simulink model "SIMULINK_02_HOMEWORK_INVERSE_IDENTIFICATION_SANTIAGO_GARCIA"  (R2020a)
settings: Solver=FixedStepAuto  StartTime=0.0  StopTime=150  FixedStep=0.01  RelTol=1e-2
libraries: simulink x1
settings Model: Creator=elkin  LastModifiedBy=USUARIO

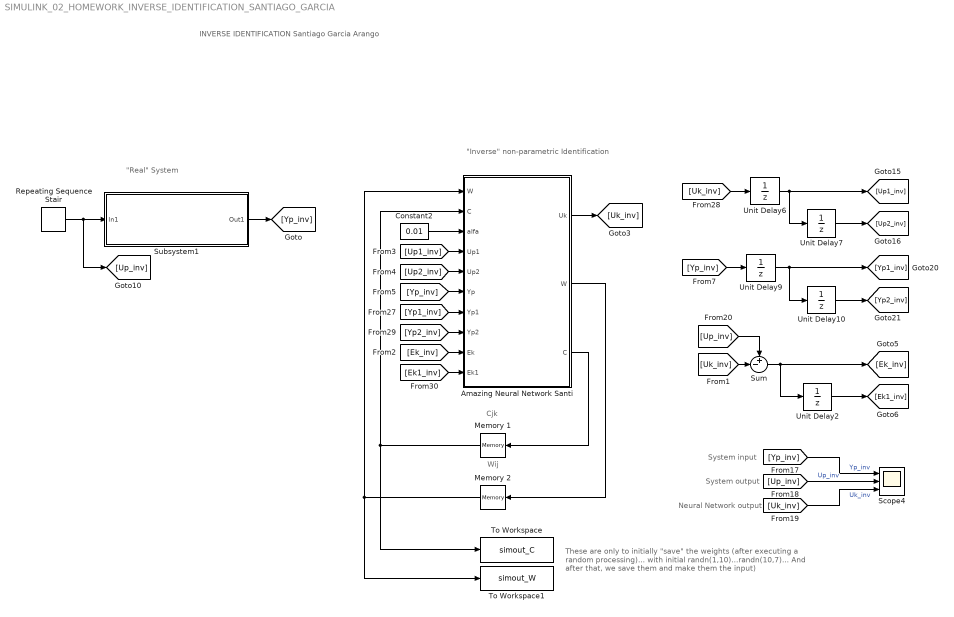
== system SIMULINK_02_HOMEWORK_INVERSE_IDENTIFICATION_SANTIAGO_GARCIA ==
  note: These are only to initially "save" the weights (after executing a random processing)... with initial randn(1,10)...randn(10,7)...
      | And after that,  we save them and make them the input)
  note: "Real" System
  note: INVERSE IDENTIFICATION
      | Santiago Garcia Arango
  note: "Inverse" non-parametric Identification
  note: Cjk
  note: Wij
  note: System input
  note: System output
  note: Neural Network output
  " Memory 2" : Memory  InitialCondition=[0.160168468969978,1.21353137879989,-1.56291773173372,0.929169980143353,0.695994193594052,-1.34686510381095,-0.289653748521687;0.421933175617497,0.436877187593544,0.666165671349512,0.137541063195606,-1.07644666007559,0.241226964817676,2.09884854078536;-0.0777054777653791,1.26008707442584,0.0176636587033483,0.0774381989337176,0.329568098519725,0.923600106862029,0.0294305745416468;-1.40499547474677,-0.342765649438291,-1.04188122704995,0.851174491843777,0.544969535049168,0.739674158347271,1.10397908720867;-0.0112601196223381,-0.768799183156363,-0.315486308406169,1.21256202395209,0.173176764089594,-0.178755445313924,-0.334973975015624;-0.556892652341610,0.141789370522390,-1.73598081128122,-0.978665689175691,0.645874102776012,-2.00118746022715,-0.989945469292243;-1.21745485974872,1.36268884465170,0.447025596332749,1.33569188423369,-1.15629544144397,-1.04648278411230,0.648907387350675;-0.0124054854051064,1.27274230512064,-0.172396006495970,-1.20850709692038,1.00898576278285,0.264634046236538,1.00048012001628;-0.195144705340148,-0.142308239828302,1.63129654132556,-1.07404750027954,0.113599563813982,0.811933866909450,1.80624743610141;0.273984746210026,-0.638527379745420,-1.35171776281153,-0.664986054870598,0.737505072399746,0.532586026418463,-0.586211714839106]
  Amazing Neural Network Santi : MATLAB Function  TreatAsAtomicUnit=on
  Constant2 : Constant  Value=0.01
  Memory 1 : Memory  InitialCondition=[-2.03120000000000,1.12670000000000,0.0650000000000000,-1.22620000000000,-0.274400000000000,-0.965500000000000,0.418700000000000,0.122100000000000,-0.0491000000000000,0.714800000000000]
  Repeating Sequence Stair : simulink/Sources/Repeating Sequence Stair  OutValues=[0 0.2 0 0.4 0.8 0.4 1].'  tsamp=15  OutMin=[]  OutMax=[]  OutDataTypeStr=double  OutputDataTypeScalingMode=double  OutDataType=fixdt(0,8)  ConRadixGroup=Best Precision: Vector-wise  OutScaling=2^-12
  Scope4 : Scope  NumInputPorts=3
  Subsystem1 : Subsystem
  Sum : Sum  Inputs=+-|
  To Workspace : ToWorkspace  VariableName=simout_C  SaveFormat=Timeseries  SampleTime=-1
  To Workspace1 : ToWorkspace  VariableName=simout_W  SaveFormat=Timeseries  SampleTime=-1
  Unit Delay{2,6..7,9..10} (5 alike) : UnitDelay  SampleTime=-1  HasFrameUpgradeWarning=on
  wires:
  Unit Delay7/1 -> [Up2_inv]
  Unit Delay6/1 -> [Up1_inv], Unit Delay7/1
  [Uk_inv] -> Unit Delay6/1
  [Yp1_inv] -> Amazing Neural Network Santi/7(Yp1)
  Amazing Neural Network Santi/2(W) -> " Memory 2"/1
  [Yp2_inv] -> Amazing Neural Network Santi/8(Yp2)
  " Memory 2"/1 -> To Workspace1/1, Amazing Neural Network Santi/1("W ")
  Amazing Neural Network Santi/3(C) -> Memory 1/1
  [Up1_inv] -> Amazing Neural Network Santi/4(Up1)
  [Up2_inv] -> Amazing Neural Network Santi/5(Up2)
  [Yp_inv] -> Amazing Neural Network Santi/6(Yp)
  Constant2/1 -> Amazing Neural Network Santi/3(alfa)
  Memory 1/1 -> To Workspace/1, Amazing Neural Network Santi/2("C ")
  [Ek1_inv] -> Amazing Neural Network Santi/10(Ek1)
  Amazing Neural Network Santi/1(Uk) -> [Uk_inv]
  [Yp_inv] -> Unit Delay9/1
  Unit Delay9/1 -> [Yp1_inv], Unit Delay10/1
  Unit Delay10/1 -> [Yp2_inv]
  Subsystem1/1(Out1) -> [Yp_inv]
  Repeating Sequence Stair/1 -> [Up_inv], Subsystem1/1(In1)
  [Up_inv] -> Scope4/2  "Up_inv"
  [Uk_inv] -> Scope4/3  "Uk_inv"
  [Yp_inv] -> Scope4/1  "Yp_inv"
  [Up_inv] -> Sum/1
  Sum/1 -> Unit Delay2/1, [Ek_inv]
  Unit Delay2/1 -> [Ek1_inv]
  [Uk_inv] -> Sum/2
  [Ek_inv] -> Amazing Neural Network Santi/9(Ek)

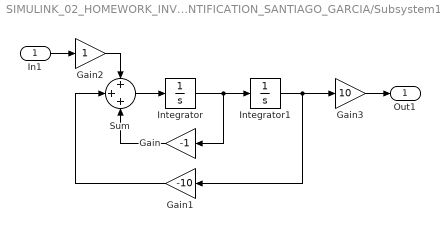
== system SIMULINK_02_HOMEWORK_INVERSE_IDENTIFICATION_SANTIAGO_GARCIA/Subsystem1 ==
  In1 : Inport
  Gain : Gain  Gain=-1
  Gain1 : Gain  Gain=-10
  Gain2 : Gain
  Gain3 : Gain  Gain=10
  Integrator : Integrator
  Integrator1 : Integrator
  Sum : Sum  Inputs=+++
  Out1 : Outport  VectorParamsAs1DForOutWhenUnconnected=off
  wires:
  Integrator/1 -> Integrator1/1, Gain/1
  Gain2/1 -> Sum/1
  Gain1/1 -> Sum/2
  Sum/1 -> Integrator/1
  Integrator1/1 -> Gain3/1, Gain1/1
  Gain/1 -> Sum/3
  In1/1 -> Gain2/1
  Gain3/1 -> Out1/1

== matlab function SIMULINK_02_HOMEWORK_INVERSE_IDENTIFICATION_SANTIAGO_GARCIA/Amazing Neural Network Santi ==
  data: W input; Uk output; C input; alfa input; Up1 input; Up2 input; Yp input; Yp1 input; Yp2 input; Ek input; W output; C output; Ek1 input
% NEURAL NETWORK FOR SIMULINK "REAL-TIME" PROCESSING BASED ON SIGNALS
% Santiago Garcia Arango
% ------------------------------------------------------------------------
% FEEDFORWARDMADALINE. Train or Test a simple neural network.
%   alfa: Learning rate constant (1 x 1)
%   W: vector of the initial Weights. size (1 x ne)
%   C: matrix of the initial hidden layers weights. size (ns x no+1)
%   REMARK: This processing is based on an "Inverse Identification"
% ------------------------------------------------------------------------

function [Uk, W, C] = fcn(W, C, alfa, Up1, Up2, Yp, Yp1, Yp2, Ek, Ek1)

activation_function_1 = "tanh";
activation_function_2 = "none";

X = [Up1 Up2 Yp Yp1 Yp2 Ek Ek1]; % Create "entries" vector
Aj = W*X'; % Add hidden layer

if (activation_function_1 == "tanh")
    H = tanh(Aj);
end

Ak = C'*H; % Add output layer

if (activation_function_2 == "none")
    Uk = Ak;
end

C = C+alfa*Ek*H; % Update weights of C

if (activation_function_1 == "tanh")
    H2 = sech(Aj).^2;
end

W = W+alfa*Ek*(C.*H2)*X; % Update weights of W

end
